simulink model "QCar2_Virtual_Car2"  (R2023a)
settings: Solver=ode1  StartTime=0.0  StopTime=inf  FixedStep=cameraStepSize/10  RelTol=1e-3  EnableMultiTasking=on
PreLoadFcn:
  | QCarSetup
values from neighbouring files (symbols this model uses):
  cameraStepSize = 3e-2    (= 0.03)    [QCarSetup.m]
  path_x = [0.826 0.836 0.846 0.856 0.866 0.876 0.886 0.896 0.906 0.916 0.926 0.936 ... (740 elements, 740x1)]    [SDTS_Paths_6_2023.mat]
  path_x2 = [-0.614 -0.604 -0.594 -0.584 -0.574 -0.564 -0.554 -0.544 -0.534 -0.524 -0.514 -0.504 ... (1090 elements, 1090x1)]    [SDTS_Paths_6_2023.mat]
  path_x3 = [-0.614 -0.603821428571 -0.593642857143 -0.583464285714 -0.573285714286 -0.563107142857 -0.552928571429 -0.54275 -0.532571428571 -0.522392857143 -0.512214285714 -0.502035714286 ... (714 elements, 714x1)]    [SDTS_Paths_6_2023.mat]
  path_x4 = [-0.614 -0.604 -0.594 -0.584 -0.574 -0.564 -0.554 -0.544 -0.534 -0.524 -0.514 -0.504 ... (1761 elements, 1761x1)]    [SDTS_Paths_6_2023.mat]
  path_x5 = [1.436 1.42588571429 1.41577142857 1.40565714286 1.39554285714 1.38542857143 1.37531428571 1.3652 1.35508571429 1.34497142857 1.33485714286 1.32474285714 ... (574 elements, 574x1)]    [SDTS_Paths_6_2023.mat]
  path_x6 = [1.436 1.42588571429 1.41577142857 1.40565714286 1.39554285714 1.38542857143 1.37531428571 1.3652 1.35508571429 1.34497142857 1.33485714286 1.32474285714 ... (1288 elements, 1288x1)]    [SDTS_Paths_6_2023.mat]
  path_y = [-1.0887 -1.0887 -1.0887 -1.0887 -1.0887 -1.0887 -1.0887 -1.0887 -1.0887 -1.0887 -1.0887 -1.0887 ... (740 elements, 740x1)]    [SDTS_Paths_6_2023.mat]
  path_y2 = [-1.0887 -1.0887 -1.0887 -1.0887 -1.0887 -1.0887 -1.0887 -1.0887 -1.0887 -1.0887 -1.0887 -1.0887 ... (1090 elements, 1090x1)]    [SDTS_Paths_6_2023.mat]
  path_y3 = [-1.0887 -1.0887 -1.0887 -1.0887 -1.0887 -1.0887 -1.0887 -1.0887 -1.0887 -1.0887 -1.0887 -1.0887 ... (714 elements, 714x1)]    [SDTS_Paths_6_2023.mat]
  path_y4 = [-1.0887 -1.0887 -1.0887 -1.0887 -1.0887 -1.0887 -1.0887 -1.0887 -1.0887 -1.0887 -1.0887 -1.0887 ... (1761 elements, 1761x1)]    [SDTS_Paths_6_2023.mat]
  path_y5 = [-0.8157 -0.8157 -0.8157 -0.8157 -0.8157 -0.8157 -0.8157 -0.8157 -0.8157 -0.8157 -0.8157 -0.8157 ... (574 elements, 574x1)]    [SDTS_Paths_6_2023.mat]
  path_y6 = [-0.8157 -0.8157 -0.8157 -0.8157 -0.8157 -0.8157 -0.8157 -0.8157 -0.8157 -0.8157 -0.8157 -0.8157 ... (1288 elements, 1288x1)]    [SDTS_Paths_6_2023.mat]
undefined symbols (not defined in the file or in its folder): DiscIntNeverNeededParam, gcbh, height, Host, JPEG, left, qc_get_step_size, top, video_display_show, width
libraries: quarc_library x71, simulink_extras x12, simulink x5
(part 1 of 5)
settings Model: SimulationMode=external  ExtModeTrigDuration=10000  Creator=user
settings SolverCC: AlgebraicLoopSolver=TrustRegion  PositivePriorityOrder=on
settings DataIOCC: ReturnWorkspaceOutputs=off
settings OptimizationCC: ReuseModelBlockBuffer=off
settings DebuggingCC: UnconnectedInputMsg=warning  UnconnectedOutputMsg=warning  UnconnectedLineMsg=warning  ArithmeticOperatorsInVariantConditions=warning
settings ModelReferenceCC: EnableRefExpFcnMdlSchedulingChecks=on
settings SFSimCC: SimUseLocalCustomCode=off  CustomCodeUndefinedFunction=UseInterfaceOnly
settings RTWCC: Description=QUARC Win64 Target Using Toolchain  SystemTargetFile=quarc_win64.tlc  TemplateMakefile=quarc_default_tmf  RTWUseLocalCustomCode=off  Toolchain=QUARC win64 | nmake (64-bit Windows)  BuildConfiguration=Faster Runs
settings CodeAppCC: StateflowObjectComments=on
settings STFCustomTargetCC: SystemTargetFile=quarc_win64.tlc
settings GRTTargetCC: ParMdlRefBuildCompliant=off  CompOptLevelCompliant=off  CombineOutputUpdateFcns=off  MatFileLogging=off  CPPClassGenCompliant=off  GRTInterface=on  ExtMode=on  ExtModeMexFile=quarc_comm
settings ConfigComp: CovMetricSettings=dswe

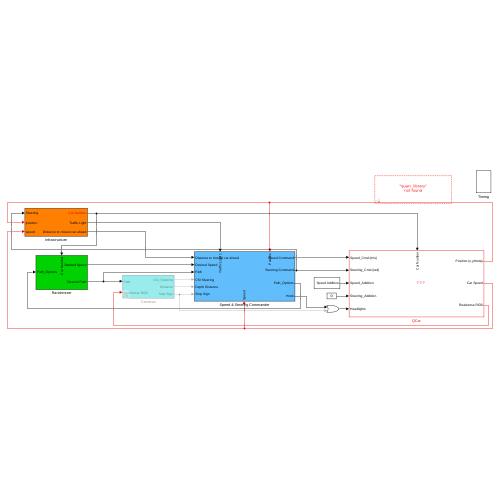
[thumbnail: Simulink's stored preview of the top-level diagram]
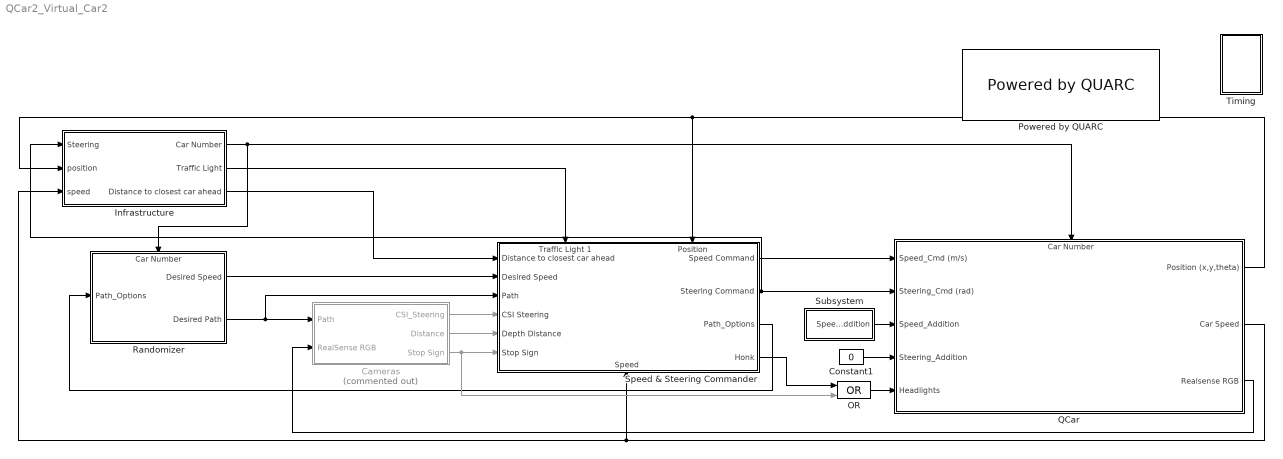
== system QCar2_Virtual_Car2 ==
  Cameras : Subsystem  Commented=on
  Constant1 : Constant  Value=0
  Infrastructure : Subsystem
  OR : Logic  Operator=OR  IconShape=distinctive  AllPortsSameDT=off  OutDataTypeStr=boolean
  Powered by QUARC : quarc_library/Logos/Powered by QUARC
  QCar : Subsystem
      settings: PortSchema="{\"entries\":[{\"content\":{\"sides\":[{\"content\":{\"connectorIds\":[\"In1\",\"In2\",\"In3\",\"In4\",\"In5\"]},\"type\":\"ConnectorPlacement.EquallySpacedRectSide\",\"uuid\":\"02a1560c-0405-4b97-a286-7d926425b90e\"},{\"content\":{\"connectorIds\":[\"Out1\",\"Out2\",\"Out3\"],\"side\":\"RIGHT\"},\"type\":\"ConnectorPlacement.EquallySpacedRectSide\",\"uuid\":\"39c5c8b2-4245-4ec7-b5b3-4c98e6a2673a\"},{\"content\":{\"connectorIds\":[\"In6\"],\"side\":\"TOP\"},\"type\":\"ConnectorPlacement.EquallySpacedRectSide\",\"uuid\":\"1752f2f8-f0ed-4d28-b225-c74112047425\"}]},\"type\":\"ConnectorPlacement.EquallySpacedConnector\",\"uuid\":\"d58cf7e2-2005-4c93-8747-d53ee0601380\"}],\"packageUris\":[\"http://schema.mathworks.com/mf0/Connector/R2020b\"],\"version\":\"1.0\"}"
      mask Display: image('QCar.png'); % Use "Edit Image" on toolstrip to change.
  Randomizer : Subsystem
      settings: PortSchema="{\"entries\":[{\"content\":{\"sides\":[{\"content\":{\"connectorIds\":[\"In1\"]},\"type\":\"ConnectorPlacement.EquallySpacedRectSide\",\"uuid\":\"79c25646-074c-450f-bb45-0d8852c7e7f6\"},{\"content\":{\"connectorIds\":[\"Out1\",\"Out2\"],\"side\":\"RIGHT\"},\"type\":\"ConnectorPlacement.EquallySpacedRectSide\",\"uuid\":\"212c2e10-164c-43b0-8e79-58f131c612df\"},{\"content\":{\"connectorIds\":[\"In2\"],\"side\":\"TOP\"},\"type\":\"ConnectorPlacement.EquallySpacedRectSide\",\"uuid\":\"61fd9557-f0fe-45db-bcdc-894cad4630c6\"}]},\"type\":\"ConnectorPlacement.EquallySpacedConnector\",\"uuid\":\"547c8944-af2b-4298-88bf-ccf6c0f693d3\"}],\"packageUris\":[\"http://schema.mathworks.com/mf0/Connector/R2020b\"],\"version\":\"1.0\"}"
  Speed & Steering Commander : Subsystem
      settings: PortSchema="{\"entries\":[{\"content\":{\"sides\":[{\"content\":{\"connectorIds\":[\"In1\",\"In2\",\"In3\",\"In4\",\"In5\",\"In6\"]},\"type\":\"ConnectorPlacement.EquallySpacedRectSide\",\"uuid\":\"9b63f585-0ce9-4b0b-9aa1-11e6ffafcd91\"},{\"content\":{\"connectorIds\":[\"Out1\",\"Out2\",\"Out3\",\"Out4\"],\"side\":\"RIGHT\"},\"type\":\"ConnectorPlacement.EquallySpacedRectSide\",\"uuid\":\"3f0be152-fc9f-4953-a169-b2152976c976\"},{\"content\":{\"connectorIds\":[\"In7\",\"In8\"],\"side\":\"TOP\"},\"type\":\"ConnectorPlacement.EquallySpacedRectSide\",\"uuid\":\"393ea782-c0f7-40ad-a810-9b99db6be290\"},{\"content\":{\"connectorIds\":[\"In9\"],\"side\":\"BOTTOM\"},\"type\":\"ConnectorPlacement.EquallySpacedRectSide\",\"uuid\":\"5db59a4e-a267-4a7e-baba-ee9e0de1ecf8\"}]},\"type\":\"ConnectorPlacement.EquallySpacedConnector\",\"uuid\":\"cc2e920a-311c-4c49-a19e-cf12c76a97eb\"}],\"packageUris\":[\"http://schema.mathworks.com/mf0/Connector/R2020b\"],\"version\":\"1.0\"}"
  Subsystem : Subsystem
  Timing : Subsystem
  wires:
  Infrastructure/2(Traffic Light) -> Speed & Steering Commander/7(Traffic Light 1)
  Speed & Steering Commander/4(Honk) -> OR/1
  OR/1 -> QCar/5(Headlights)
  QCar/3(Realsense RGB) -> Cameras/2(RealSense RGB)
  QCar/2(Car Speed) -> Infrastructure/3("speed "), Speed & Steering Commander/9(Speed)
  Speed & Steering Commander/3(Path_Options) -> Randomizer/1(Path_Options)
  Cameras/3(Stop Sign) -> OR/2, Speed & Steering Commander/6(Stop Sign)
  Randomizer/2(Desired Path) -> Speed & Steering Commander/3(Path), Cameras/1(Path)
  Infrastructure/1(Car Number) -> QCar/6(Car Number), Randomizer/2(Car Number)
  Cameras/2(Distance) -> Speed & Steering Commander/5(Depth Distance)
  Speed & Steering Commander/1(Speed Command) -> QCar/1(Speed_Cmd (m/s))
  QCar/1(Position (x,y,theta)) -> Speed & Steering Commander/8(Position), Infrastructure/2(position)
  Infrastructure/3(Distance to closest car ahead) -> Speed & Steering Commander/1(Distance to closest car ahead)
  Cameras/1(CSI_Steering) -> Speed & Steering Commander/4(CSI Steering)
  Speed & Steering Commander/2(Steering Command) -> Infrastructure/1(Steering), QCar/2(Steering_Cmd (rad))
  Constant1/1 -> QCar/4(Steering_Addition)
  Randomizer/1(Desired Speed) -> Speed & Steering Commander/2(Desired Speed)
  Subsystem/1(Speed Addition) -> QCar/3(Speed_Addition)

== system QCar2_Virtual_Car2/Cameras ==
  Path : Inport
  RealSense RGB : Inport  Port=2
  CSI Camera : Subsystem  Commented=on
  Classifier : Scope
  Demux : Demux  Outputs=5
  Goto : Goto  Commented=on  GotoTag=CSI_Steering
  Goto1 : Goto  Commented=on  GotoTag=CSI_Score
  Goto23 : Goto  Commented=on  GotoTag=Found_Lane
  Goto24 : Goto  Commented=on  GotoTag=Lost_Lane
  Image Transform : quarc_library/Image Processing/Generic/Image Transform  algorithm=Resize  color_theme=KRYGCBMW  min_pixel=0  max_pixel=4000  contour_depth=1  focal_length=308  principal_point=[262 334]  radial_coeffs=[-0.3129 0.0907]  tangential_coeffs=[]  extrapolated_pixel=0  interpolation=nearest  row_coords=0  column_coords=0  output_height=224  output_width=224  angle=0  origin=[240 320]  output_origin=[240 320]  output_data_type=uint8
      settings: AttributesFormatString=(%<algorithm>)  SourceProductName=QUARC Targets
  Rate Transition : RateTransition
  Real Sense : Subsystem  LoadFcn=set_param(gcbh, 'UserData', gcb);  StartFcn=video_display_show([gcb, '/Video Display'], 'add', gcb);  mask(Video Compressed Display){algorithm=JPEG, quality=50, sample_time=-1, use_hardware=on}
      mask prompts: algorithm "Compression algorithm:"; quality "Compression quality (0-100):"; sample_time "Sample time (seconds):"; use_hardware "Use hardware acceleration for video display"
      mask help: Displays a video stream on the host, using compression to minimize bandwidth.
      mask init:
      | qc_set_display('Video\nCompressed\nDisplay');
      settings: UndoDeleteFcn=set_param(gcbh, 'UserData', gcb);  OpenFcn=video_display_show([gcb, '/Video Display'], 'show', gcb);  PreDeleteFcn=video_display_show([gcb, '/Video Display'], 'delete');
      settings: CopyFcn=|
      | set_param(gcbh, 'UserData', gcb);
      | set_param(gcbh, 'LinkStatus', 'none');
      settings: NameChangeFcn=|
      | video_display_show([get_param(gcbh, 'UserData'), '/Video Display'], 'rename', [gcb, '/Video Display']);
      | video_display_show([gcb, '/Video Display'], 'add', gcb);
      | set_param(gcbh, 'UserData', gcb);
      mask Help: web(qc_get_block_help_path(gcb));
      mask TypeOptions algorithm: Image Compress/algorithm
      mask TypeOptions quality: Image Compress/quality
      mask TypeOptions sample_time: Video Display/sample_time
      mask TypeOptions use_hardware: Video Display/use_hardware
      mask Display:
      | patch([0.98591 0.98591 0.62618 0.59072 0.56147   0.536   0.536  0.5441 0.56912 0.59207 0.60881 0.62276 0.63527 0.64364  0.6485  0.6485 0.64706 0.64499 0.63662 0.62411 0.61232 0.59837 0.58307 0.56147   0.536   0.536  0.5441  0.5747 0.60953 0.63662 0.67001  0.7034 0.72851 0.75425 0.77927 0.80294 0.82454 0.84119 0.85865 0.87395 0.88574 0.89339  0.8969 0.89969 0.89969 0.89267  0.8816 0.87044 0.85649  0.8384 0.81824 0.80294 0.78764 0.77513 0.76676 0.75776 0.76397 0.77513 0.79178 0.80987 0.82796 0.84326 0.86207 0.98528],[0.18689 0.05522 0.05522 0.05171 0.05171    0.05 0.18338 0.18338 0.19148 0.20435 0.22298 0.24863 0.28589 0.33125 0.38138 0.55139 0.59801 0.63761 0.68189 0.72149 0.74939 0.76694 0.77855 0.79367 0.79952 0.92768 0.92768 0.92768 0.92417 0.92066 0.91364  0.9032 0.89384 0.88106 0.86594 0.85073 0.82634 0.80537 0.77855 0.74363 0.70403 0.65858 0.61079 0.59099 0.41513 0.37202 0.31847 0.29048 0.25556 0.23342  0.2102 0.19382 0.18221 0.17285 0.16943 0.16124  0.1589 0.16241 0.16709 0.17168  0.1787 0.18221 0.18689 0.18689],[0.9,0.90,0.91])
      | patch([0.536 0.52601 0.46823 0.44528 0.41603 0.39101 0.35555 0.33116 0.31451 0.29291  0.2804 0.26717 0.25322 0.23999 0.22406 0.20732 0.19337 0.17528 0.15935 0.14396 0.13217 0.11759 0.10922 0.10085 0.09671 0.09392 0.09041 0.08906 0.08906 0.09464  0.0995 0.10778 0.11894 0.13145 0.14675 0.16349 0.17672 0.19409 0.20732 0.22406 0.23999 0.26159 0.27833 0.29849 0.31793 0.33602 0.35411 0.37085 0.39245 0.41603   0.536   0.536 0.53159 0.46409   0.446 0.42026 0.39587 0.37571 0.36113 0.34925 0.34088 0.33809 0.33809 0.34088 0.34583 0.35627 0.36392 0.38129 0.39587 0.41117 0.42719 0.44672  0.4676 0.48353 0.48353 0.52394   0.536],[0.05 0.04829 0.04712 0.04712 0.04829 0.05063 0.05405 0.05873 0.06107 0.06692 0.07043 0.07619 0.08087 0.08672 0.09482 0.10652 0.11696 0.13325  0.1508 0.17168 0.19499 0.22415 0.25439 0.28472 0.31379 0.35456 0.38489 0.41513 0.58055 0.63878 0.68774 0.72149 0.75641 0.78089 0.80537 0.82859 0.84029 0.85658 0.86594 0.87404  0.8834 0.89267 0.90086 0.90788 0.91247 0.91832 0.92066   0.923 0.92651 0.92768 0.92768 0.79952 0.79952 0.79952 0.79718 0.78899 0.77153 0.75056 0.72149 0.68072 0.62249  0.5549 0.41396 0.37085 0.33242 0.28121 0.25205 0.22181 0.20552 0.19499 0.18572 0.18221 0.17753 0.17636 0.17753  0.1787  0.1787],[0.9,0.90,0.91])
      | disp('Video\nCompressed\nDisplay');
  S-Function : S-Function  Commented=on  FunctionName=classify_image_caller  SFunctionDeploymentMode=off  EnableBusSupport=off
  Selector : Selector  NumberOfDimensions=3  InputPortWidth=3  IndexOptions=Select all,Index vector (dialog),Select all  Indices=[1 3],140:499,1  OutputSizes=1,1,1
  Sign Finder : Subsystem
  Sign ROI : Subsystem  LoadFcn=set_param(gcbh, 'UserData', gcb);  StartFcn=video_display_show([gcb, '/Video Display'], 'add', gcb);  mask(Video Compressed Display){algorithm=JPEG, quality=50, sample_time=-1, use_hardware=on}
      mask prompts: algorithm "Compression algorithm:"; quality "Compression quality (0-100):"; sample_time "Sample time (seconds):"; use_hardware "Use hardware acceleration for video display"
      mask help: Displays a video stream on the host, using compression to minimize bandwidth.
      mask init:
      | qc_set_display('Video\nCompressed\nDisplay');
      settings: UndoDeleteFcn=set_param(gcbh, 'UserData', gcb);  OpenFcn=video_display_show([gcb, '/Video Display'], 'show', gcb);  PreDeleteFcn=video_display_show([gcb, '/Video Display'], 'delete');
      settings: CopyFcn=|
      | set_param(gcbh, 'UserData', gcb);
      | set_param(gcbh, 'LinkStatus', 'none');
      settings: NameChangeFcn=|
      | video_display_show([get_param(gcbh, 'UserData'), '/Video Display'], 'rename', [gcb, '/Video Display']);
      | video_display_show([gcb, '/Video Display'], 'add', gcb);
      | set_param(gcbh, 'UserData', gcb);
      mask Help: web(qc_get_block_help_path(gcb));
      mask TypeOptions algorithm: Image Compress/algorithm
      mask TypeOptions quality: Image Compress/quality
      mask TypeOptions sample_time: Video Display/sample_time
      mask TypeOptions use_hardware: Video Display/use_hardware
      mask Display:
      | patch([0.98591 0.98591 0.62618 0.59072 0.56147   0.536   0.536  0.5441 0.56912 0.59207 0.60881 0.62276 0.63527 0.64364  0.6485  0.6485 0.64706 0.64499 0.63662 0.62411 0.61232 0.59837 0.58307 0.56147   0.536   0.536  0.5441  0.5747 0.60953 0.63662 0.67001  0.7034 0.72851 0.75425 0.77927 0.80294 0.82454 0.84119 0.85865 0.87395 0.88574 0.89339  0.8969 0.89969 0.89969 0.89267  0.8816 0.87044 0.85649  0.8384 0.81824 0.80294 0.78764 0.77513 0.76676 0.75776 0.76397 0.77513 0.79178 0.80987 0.82796 0.84326 0.86207 0.98528],[0.18689 0.05522 0.05522 0.05171 0.05171    0.05 0.18338 0.18338 0.19148 0.20435 0.22298 0.24863 0.28589 0.33125 0.38138 0.55139 0.59801 0.63761 0.68189 0.72149 0.74939 0.76694 0.77855 0.79367 0.79952 0.92768 0.92768 0.92768 0.92417 0.92066 0.91364  0.9032 0.89384 0.88106 0.86594 0.85073 0.82634 0.80537 0.77855 0.74363 0.70403 0.65858 0.61079 0.59099 0.41513 0.37202 0.31847 0.29048 0.25556 0.23342  0.2102 0.19382 0.18221 0.17285 0.16943 0.16124  0.1589 0.16241 0.16709 0.17168  0.1787 0.18221 0.18689 0.18689],[0.9,0.90,0.91])
      | patch([0.536 0.52601 0.46823 0.44528 0.41603 0.39101 0.35555 0.33116 0.31451 0.29291  0.2804 0.26717 0.25322 0.23999 0.22406 0.20732 0.19337 0.17528 0.15935 0.14396 0.13217 0.11759 0.10922 0.10085 0.09671 0.09392 0.09041 0.08906 0.08906 0.09464  0.0995 0.10778 0.11894 0.13145 0.14675 0.16349 0.17672 0.19409 0.20732 0.22406 0.23999 0.26159 0.27833 0.29849 0.31793 0.33602 0.35411 0.37085 0.39245 0.41603   0.536   0.536 0.53159 0.46409   0.446 0.42026 0.39587 0.37571 0.36113 0.34925 0.34088 0.33809 0.33809 0.34088 0.34583 0.35627 0.36392 0.38129 0.39587 0.41117 0.42719 0.44672  0.4676 0.48353 0.48353 0.52394   0.536],[0.05 0.04829 0.04712 0.04712 0.04829 0.05063 0.05405 0.05873 0.06107 0.06692 0.07043 0.07619 0.08087 0.08672 0.09482 0.10652 0.11696 0.13325  0.1508 0.17168 0.19499 0.22415 0.25439 0.28472 0.31379 0.35456 0.38489 0.41513 0.58055 0.63878 0.68774 0.72149 0.75641 0.78089 0.80537 0.82859 0.84029 0.85658 0.86594 0.87404  0.8834 0.89267 0.90086 0.90788 0.91247 0.91832 0.92066   0.923 0.92651 0.92768 0.92768 0.79952 0.79952 0.79952 0.79718 0.78899 0.77153 0.75056 0.72149 0.68072 0.62249  0.5549 0.41396 0.37085 0.33242 0.28121 0.25205 0.22181 0.20552 0.19499 0.18572 0.18221 0.17753 0.17636 0.17753  0.1787  0.1787],[0.9,0.90,0.91])
      | disp('Video\nCompressed\nDisplay');
  Stop : Scope
  Stop1 : Scope
  CSI_Steering : Outport
  Distance : Outport  Port=2
  Stop Sign : Outport  Port=3
  wires:
  Selector/1 -> Image Transform/1
  Sign Finder/1(Stop Sign) -> Stop/1, Stop Sign/1
  Demux/4 -> Stop1/1
  RealSense RGB/1 -> Selector/1, Real Sense/1(In1)
  S-Function/1 -> Rate Transition/1, Classifier/1, Demux/1
  Image Transform/1 -> S-Function/1, Sign ROI/1(In1)
  Rate Transition/1 -> Sign Finder/1(Signs)
  CSI Camera/3(Found Lane) -> Goto23/1
  CSI Camera/1(Steering) -> Goto/1, CSI_Steering/1
  CSI Camera/2(Score) -> Goto1/1
  CSI Camera/4(Lost Lane) -> Goto24/1

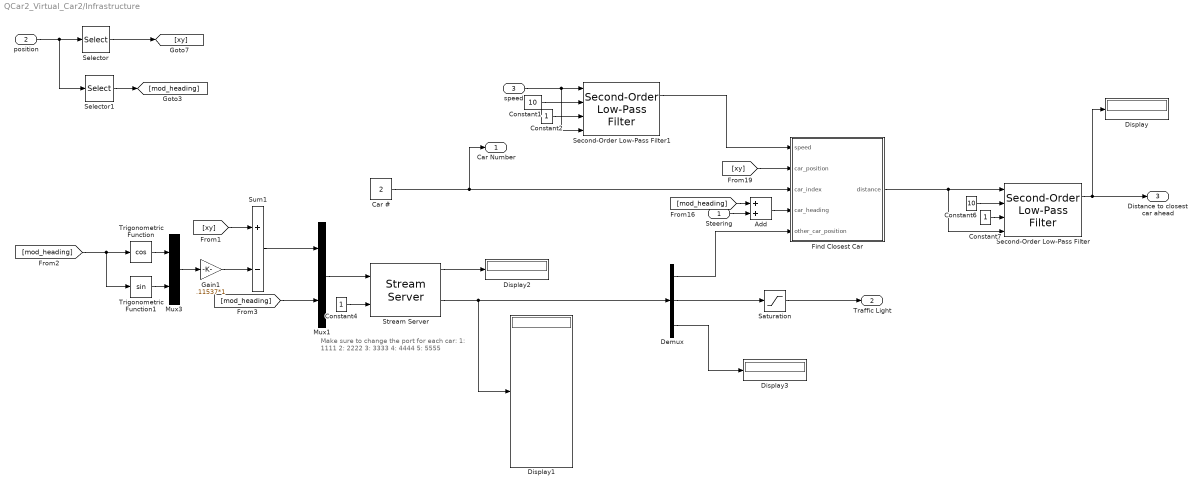
== system QCar2_Virtual_Car2/Infrastructure ==
  note: Make sure to change the port for each car:
      | 1: 1111
      | 2: 2222
      | 3: 3333
      | 4: 4444
      | 5: 5555
  Steering : Inport
  position : Inport  Port=2
  "speed " : Inport  Port=3
  Add : Sum
  Car # : Constant  Value=2
  Constant1 : Constant  Value=10
  Constant2 : Constant
  Constant4 : Constant
  Constant6 : Constant  Value=10
  Constant7 : Constant
  Demux : Demux  Outputs=[10 1 1]
  Display{,1..3} (4 alike) : Display
      Display2 settings: Decimation=100
      Display3 settings: Decimation=100
  Find Closest Car : Subsystem
  Gain1 : Gain  Gain=.11537*1
  Mux1 : Mux  Inputs=2
  Mux3 : Mux  Inputs=2
  Saturation : Saturate  UpperLimit=1  LowerLimit=0
  Second-Order Low-Pass Filter : quarc_library/Continuous/Second-Order Low-Pass Filter  params_source=External (input ports)  input_width=1  input_zeta=1  input_init=0
  Second-Order Low-Pass Filter1 : quarc_library/Continuous/Second-Order Low-Pass Filter  params_source=External (input ports)  input_width=1  input_zeta=1  input_init=0
  Selector : Selector  InputPortWidth=3  IndexOptions=Index vector (dialog)  Indices=1:2  OutputSizes=1
  Selector1 : Selector  InputPortWidth=3  IndexOptions=Index vector (dialog)  Indices=3  OutputSizes=1
  Stream Server : quarc_library/Communications/Basic/Stream Server  uri_source=Specify via dialog (do not evaluate)  uri=tcpip://localhost:2222  send_buffer_size=1460  receive_buffer_size=1460  byte_order=little endian (Intel - LSB first)  optimization=Minimum latency  send_options=Send most recent data  receive_options=Receive most recent data  default_value=10* ones (1,12)  sample_time=qc_get_step_size  active=off  implementation=Use blocking I/O in a separate thread  send_fifo_size=1000  receive_fifo_size=1000  send_priority=0  receive_priority=0  send_dimensions=off  receive_dimensions=off  max_dimensions=-1  data_type=Inherited via back propagation  type_expr=BusObject
      settings: AttributesFormatString="\"tcpip://localhost:2222\""
  Sum1 : Sum  Inputs=+-
  Trigonometric Function : Trigonometry  Operator=cos
  Trigonometric Function1 : Trigonometry
  Car Number : Outport
  Traffic Light : Outport  Port=2
  Distance to closest car ahead : Outport  Port=3
  wires:
  Mux1/1 -> Stream Server/1
  [xy] -> Sum1/1
  Mux3/1 -> Gain1/1
  Trigonometric Function1/1 -> Mux3/2
  Trigonometric Function/1 -> Mux3/1
  Gain1/1 -> Sum1/2
  Saturation/1 -> Traffic Light/1
  Demux/2 -> Saturation/1
  Demux/1 -> Find Closest Car/5(other_car_position)
  Steering/1 -> Add/2
  [mod_heading] -> Add/1
  Add/1 -> Find Closest Car/4(car_heading)
  Find Closest Car/1(distance) -> Second-Order Low-Pass Filter/1, Second-Order Low-Pass Filter/4
  Second-Order Low-Pass Filter1/1 -> Find Closest Car/1("speed ")
  Constant2/1 -> Second-Order Low-Pass Filter1/3
  [xy] -> Find Closest Car/2(car_position)
  "speed "/1 -> Second-Order Low-Pass Filter1/1, Second-Order Low-Pass Filter1/4
  Car #/1 -> Car Number/1, Find Closest Car/3(car_index)
  Constant1/1 -> Second-Order Low-Pass Filter1/2
  Second-Order Low-Pass Filter/1 -> Distance to closest car ahead/1, Display/1
  Selector1/1 -> [mod_heading]
  Selector/1 -> [xy]
  position/1 -> Selector/1, Selector1/1
  Constant6/1 -> Second-Order Low-Pass Filter/2
  Constant4/1 -> Stream Server/2
  Constant7/1 -> Second-Order Low-Pass Filter/3
  Stream Server/1 -> Display2/1
  Stream Server/4 -> Display1/1, Demux/1
  Sum1/1 -> Mux1/1
  [mod_heading] -> Mux1/2
  [mod_heading] -> Trigonometric Function1/1, Trigonometric Function/1
  Demux/3 -> Display3/1

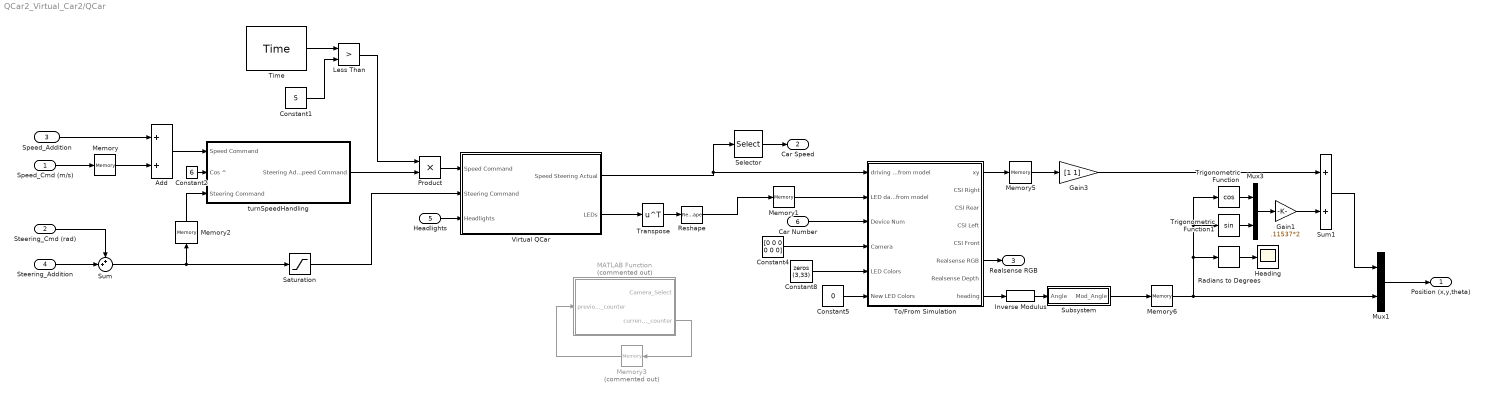
== system QCar2_Virtual_Car2/QCar ==
  Speed_Cmd (m/s) : Inport
  Steering_Cmd (rad) : Inport  Port=2
  Speed_Addition : Inport  Port=3
  Steering_Addition : Inport  Port=4
  Headlights : Inport  Port=5
  Car Number : Inport  Port=6
  Add : Sum
  Constant1 : Constant  Value=5
  Constant2 : Constant  Value=6
  Constant4 : Constant  Value=[0 0 0 0 0 0]
  Constant5 : Constant  Value=0
  Constant8 : Constant  Value=zeros (3,33)
  Gain1 : Gain  Gain=.11537*2
  Gain3 : Gain  Gain=[1 1]
  Heading : Scope
  Inverse Modulus : quarc_library/Discontinuities/Inverse Modulus  modulus=2*pi  output_derivative=off  output_revolutions=off  max_x=Inf  min_x=-Inf
  Less Than : RelationalOperator  Operator=>  OutDataTypeStr=boolean  RndMeth=Simplest  InputSameDT=off
  MATLAB Function : MATLAB Function  Commented=on  TreatAsAtomicUnit=on
  Memory : Memory  InheritSampleTime=on  LinearizeMemory=on  LinearizeAsDelay=on
  Memory1 : Memory  InitialCondition=zeros (1,16)  InheritSampleTime=on  LinearizeMemory=on  LinearizeAsDelay=on
  Memory2 : Memory  InheritSampleTime=on  LinearizeMemory=on  LinearizeAsDelay=on
  Memory3 : Memory  Commented=on  InheritSampleTime=on  LinearizeMemory=on  LinearizeAsDelay=on
  Memory5 : Memory  InitialCondition=[0 0]  InheritSampleTime=on  LinearizeMemory=on  LinearizeAsDelay=on
  Memory6 : Memory  InheritSampleTime=on  LinearizeMemory=on  LinearizeAsDelay=on
  Mux1 : Mux  Inputs=2
  Mux3 : Mux  Inputs=2
  Product : Product
  Radians to Degrees : simulink_extras/Transformations/Radians to Degrees
  Reshape : Reshape
  Saturation : Saturate  UpperLimit=0.6  LowerLimit=-0.6
  Selector : Selector  InputPortWidth=2  IndexOptions=Index vector (dialog)  Indices=[1]  OutputSizes=1
  Subsystem : Subsystem
  Sum : Sum  Inputs=++|
  Sum1 : Sum
  Time : quarc_library/Sources/Time/Time  time_source=Wall clock  sample_time=qc_get_step_size
  To/From Simulation : Subsystem
  Transpose : Math  Operator=transpose
  Trigonometric Function : Trigonometry  Operator=cos
  Trigonometric Function1 : Trigonometry
  Virtual QCar : Subsystem
  turnSpeedHandling : Subsystem
  Position (x,y,theta) : Outport
  Car Speed : Outport  Port=2
  Realsense RGB : Outport  Port=3
  wires:
  Saturation/1 -> Virtual QCar/2(Steering Command)
  Memory6/1 -> Mux1/2, Trigonometric Function/1, Trigonometric Function1/1, Radians to Degrees/1
  Subsystem/1(Mod_Angle) -> Memory6/1
  Memory5/1 -> Gain3/1
  Headlights/1 -> Virtual QCar/3(Headlights)
  Memory3/1 -> MATLAB Function/1(previous_counter)
  MATLAB Function/2(current_counter) -> Memory3/1
  Mux1/1 -> Position (x,y,theta)/1
  Sum1/1 -> Mux1/1
  Memory2/1 -> turnSpeedHandling/3(Steering Command)
  Add/1 -> turnSpeedHandling/1(Speed Command)
  Constant2/1 -> turnSpeedHandling/2(Cos ^)
  Car Number/1 -> To/From Simulation/3(Device Num)
  Gain3/1 -> Sum1/1
  Gain1/1 -> Sum1/2
  Mux3/1 -> Gain1/1
  Trigonometric Function1/1 -> Mux3/2
  Trigonometric Function/1 -> Mux3/1
  Sum/1 -> Saturation/1, Memory2/1
  Steering_Addition/1 -> Sum/2
  Radians to Degrees/1 -> Heading/1
  Memory/1 -> Add/2
  Steering_Cmd (rad)/1 -> Sum/1
  Speed_Cmd (m/s)/1 -> Memory/1
  Speed_Addition/1 -> Add/1
  Inverse Modulus/1 -> Subsystem/1(Angle)
  Virtual QCar/1(Speed Steering Actual) -> Selector/1, To/From Simulation/1(driving data from model)
  Selector/1 -> Car Speed/1
  Constant4/1 -> To/From Simulation/4(Camera)
  Constant8/1 -> To/From Simulation/5(LED Colors)
  Constant5/1 -> To/From Simulation/6(New LED Colors)
  To/From Simulation/8(heading) -> Inverse Modulus/1
  To/From Simulation/1(xy) -> Memory5/1
  To/From Simulation/6(Realsense RGB) -> Realsense RGB/1
  Memory1/1 -> To/From Simulation/2(LED data from model)
  Virtual QCar/2(LEDs) -> Transpose/1
  Transpose/1 -> Reshape/1
  Reshape/1 -> Memory1/1
  Time/1 -> Less Than/1
  Constant1/1 -> Less Than/2
  Less Than/1 -> Product/1
  Product/1 -> Virtual QCar/1(Speed Command)
  turnSpeedHandling/1(Steering Adjusted Speed Command) -> Product/2

== system QCar2_Virtual_Car2/Randomizer ==
  Path_Options : Inport
  Car Number : Inport  Port=2
  Constant1 : Constant  Value=.75
  Constant2 : Constant
  Constant3 : Constant  Value=2
  Constant4 : Constant  Value=2
  Constant5 : Constant  Value=0.7
  Constant6 : Constant  Value=0.4
  Constant7 : Constant  Value=0
  Display : Display
  Display1 : Display
  Display2 : Display
  MATLAB Function : MATLAB Function  TreatAsAtomicUnit=on
  Manual Switch : ManualSwitch
  Manual Switch1 : ManualSwitch
  Manual Switch2 : ManualSwitch
  Memory1 : Memory  InitialCondition=2  InheritSampleTime=on  LinearizeMemory=on  LinearizeAsDelay=on
  Memory2 : Memory  InitialCondition=1  InheritSampleTime=on  LinearizeMemory=on  LinearizeAsDelay=on
  Multiport Switch : MultiPortSwitch  SaturateOnIntegerOverflow=off  InputSameDT=off
  Subsystem1 : Subsystem
  Desired Speed : Outport
  Desired Path : Outport  Port=2
  wires:
  Path_Options/1 -> MATLAB Function/3(Path_Options), Display2/1
  Manual Switch2/1 -> Desired Path/1
  Constant4/1 -> Manual Switch2/2
  Manual Switch/1 -> MATLAB Function/4(Speed_Cmd_Base)
  Constant1/1 -> Manual Switch/1
  Subsystem1/1(RisingEdgeTrigger) -> MATLAB Function/5(randomize)
  Constant3/1 -> Subsystem1/1(Random Period)
  MATLAB Function/2(Desired_Speed) -> Display1/1, Memory2/1
  MATLAB Function/1(Desired_Path) -> Display/1, Manual Switch2/1, Memory1/1
  Memory2/1 -> MATLAB Function/2(Previous_Speed)
  Memory1/1 -> MATLAB Function/1(Previous_Path)
  Car Number/1 -> Multiport Switch/1
  Constant2/1 -> Multiport Switch/2
  Constant5/1 -> Multiport Switch/3
  Constant6/1 -> Multiport Switch/4
  Multiport Switch/1 -> Manual Switch1/1
  Manual Switch1/1 -> Desired Speed/1
  Constant7/1 -> Manual Switch1/2

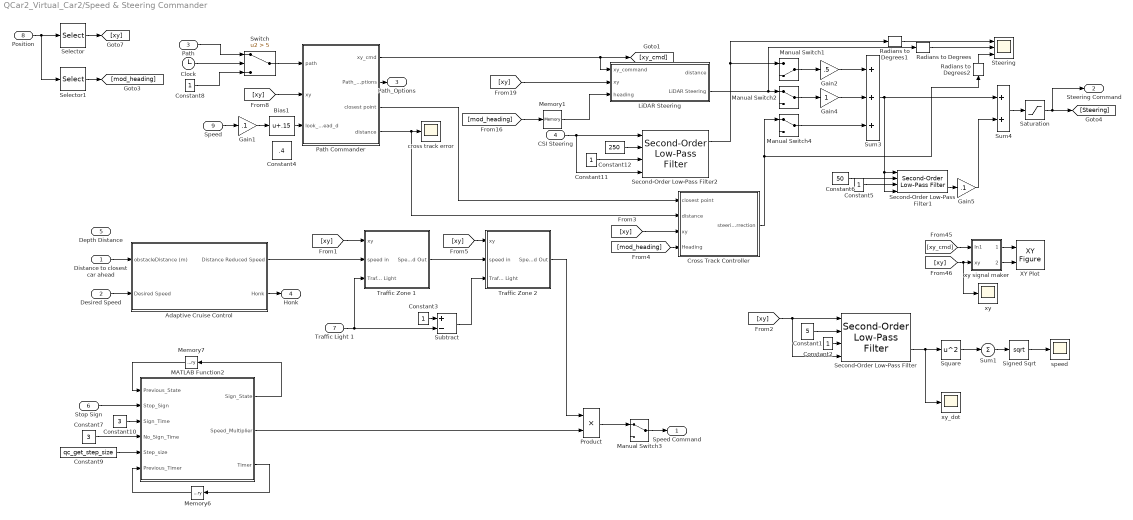
== system QCar2_Virtual_Car2/Speed & Steering Commander ==
  Distance to closest car ahead : Inport
  Desired Speed : Inport  Port=2
  Path : Inport  Port=3
  CSI Steering : Inport  Port=4
  Depth Distance : Inport  Port=5
  Stop Sign : Inport  Port=6
  Traffic Light 1 : Inport  Port=7
  Position : Inport  Port=8
  Speed : Inport  Port=9
  Adaptive Cruise Control : Subsystem
  Bias1 : Bias  Bias=.15  SaturateOnIntegerOverflow=off
  Clock : Clock
  Constant1 : Constant  Value=5
  Constant10 : Constant  Value=3
  Constant{2..3,5,8,11} (5 alike) : Constant
  Constant12 : Constant  Value=250
  Constant4 : Constant  Value=.4
  Constant6 : Constant  Value=50
  Constant7 : Constant  Value=3
  Constant9 : Constant  Value=qc_get_step_size
  Cross Track Controller : Subsystem
  Gain1 : Gain  Gain=.1
  Gain2 : Gain  Gain=.5
  Gain4 : Gain
  Gain5 : Gain  Gain=.1
  LiDAR Steering : Subsystem
  MATLAB Function2 : MATLAB Function  TreatAsAtomicUnit=on
  Manual Switch1 : ManualSwitch  CurrentSetting=0
  Manual Switch2 : ManualSwitch
  Manual Switch3 : ManualSwitch
  Manual Switch4 : ManualSwitch
  Memory1 : Memory
  Memory6 : Memory  InheritSampleTime=on  LinearizeMemory=on  LinearizeAsDelay=on
  Memory7 : Memory  InitialCondition=1  InheritSampleTime=on  LinearizeMemory=on  LinearizeAsDelay=on
  Path Commander : Subsystem
  Product : Product
  Radians to Degrees : simulink_extras/Transformations/Radians to Degrees
  Radians to Degrees1 : simulink_extras/Transformations/Radians to Degrees
  Radians to Degrees2 : simulink_extras/Transformations/Radians to Degrees
  Saturation : Saturate  UpperLimit=.6  LowerLimit=-0.6
  Second-Order Low-Pass Filter : quarc_library/Continuous/Second-Order Low-Pass Filter  params_source=External (input ports)  input_width=1  input_zeta=1  input_init=0
  Second-Order Low-Pass Filter1 : quarc_library/Continuous/Second-Order Low-Pass Filter  params_source=External (input ports)  input_width=1  input_zeta=1  input_init=0
  Second-Order Low-Pass Filter2 : quarc_library/Continuous/Second-Order Low-Pass Filter  params_source=External (input ports)  input_width=1  input_zeta=1  input_init=0
  Selector : Selector  InputPortWidth=3  IndexOptions=Index vector (dialog)  Indices=1:2  OutputSizes=1
  Selector1 : Selector  InputPortWidth=3  IndexOptions=Index vector (dialog)  Indices=3  OutputSizes=1
  Signed Sqrt : Sqrt
  Square : Math  Operator=square
  Steering : Scope  NumInputPorts=3
  Subtract : Sum  Inputs=+-
  Sum1 : Sum  Inputs=+
  Sum3 : Sum  Inputs=+++
  Sum4 : Sum
  Switch : Switch  Criteria=u2 > Threshold  Threshold=5  SaturateOnIntegerOverflow=off  InputSameDT=off
  Traffic Zone 1 : Subsystem
  Traffic Zone 2 : Subsystem
  XY Plot : quarc_library/Sinks/Figures/XY Figure  figure_mode=Use figure window  figure_tag=figure1  axes_tag=axes1  plot_mode=Time-based  minimum_x=-5  maximum_x=5  minimum_y=-2  maximum_y=5  buffer_size=1e3  update_rate=20  initial_position="1922     2   958  1021"  initial_visibility=on  sample_time=-1
      settings: SourceProductName=QUARC Targets
  cross track error : Scope
  speed : Scope
  xy : Scope
  xy signal maker : Subsystem
  xy_dot : Scope
  Speed Command : Outport
  Steering Command : Outport  Port=2
  Path_Options : Outport  Port=3
  Honk : Outport  Port=4
  wires:
  Memory1/1 -> LiDAR Steering/3(heading)
  [xy] -> LiDAR Steering/2(xy)
  Adaptive Cruise Control/2(Honk) -> Honk/1
  Constant3/1 -> Subtract/1
  Traffic Zone 2/1(Speed Out) -> Product/1
  Traffic Zone 1/1(Speed Out) -> Traffic Zone 2/2(speed in)
  [xy] -> Traffic Zone 2/1(xy)
  Adaptive Cruise Control/1(Distance Reduced Speed) -> Traffic Zone 1/2(speed in)
  Path Commander/4(distance) -> Cross Track Controller/2(distance), cross track error/1
  Cross Track Controller/1(steering correction) -> Manual Switch4/1, Radians to Degrees2/1
  Manual Switch4/1 -> Sum3/3
  [mod_heading] -> Cross Track Controller/4(Heading)
  [xy] -> Cross Track Controller/3(xy)
  Path Commander/3(closest point) -> Cross Track Controller/1(closest point)
  Manual Switch3/1 -> Speed Command/1
  Product/1 -> Manual Switch3/1
  [xy] -> Traffic Zone 1/1(xy)
  Constant12/1 -> Second-Order Low-Pass Filter2/2
  Constant11/1 -> Second-Order Low-Pass Filter2/3
  Second-Order Low-Pass Filter2/1 -> Manual Switch1/1, Radians to Degrees1/1
  CSI Steering/1 -> Second-Order Low-Pass Filter2/4, Second-Order Low-Pass Filter2/1
  Radians to Degrees2/1 -> Steering/3
  Radians to Degrees1/1 -> Steering/1
  Radians to Degrees/1 -> Steering/2
  LiDAR Steering/2(LiDAR Steering) -> Manual Switch2/1, Radians to Degrees/1
  Manual Switch2/1 -> Gain4/1
  Manual Switch1/1 -> Gain2/1
  Square/1 -> Sum1/1
  Second-Order Low-Pass Filter/2 -> Square/1, xy_dot/1
  [xy] -> xy signal maker/2(xy), xy/1
  xy signal maker/1(Out1) -> XY Plot/1
  Constant1/1 -> Second-Order Low-Pass Filter/2
  Signed Sqrt/1 -> speed/1
  Sum1/1 -> Signed Sqrt/1
  [xy_cmd] -> xy signal maker/1(In1)
  Constant2/1 -> Second-Order Low-Pass Filter/3
  [xy] -> Second-Order Low-Pass Filter/1, Second-Order Low-Pass Filter/4
  xy signal maker/2(Out2) -> XY Plot/2
  Saturation/1 -> [Steering], Steering Command/1
  Stop Sign/1 -> MATLAB Function2/2(Stop_Sign)
  Constant10/1 -> MATLAB Function2/3(Sign_Time)
  MATLAB Function2/2(Speed_Multiplier) -> Product/2
  Memory6/1 -> MATLAB Function2/6(Previous_Timer)
  Constant7/1 -> MATLAB Function2/4(No_Sign_Time)
  MATLAB Function2/1(Sign_State) -> Memory7/1
  MATLAB Function2/3(Timer) -> Memory6/1
  Memory7/1 -> MATLAB Function2/1(Previous_State)
  Constant9/1 -> MATLAB Function2/5(Step_size)
  Desired Speed/1 -> Adaptive Cruise Control/2(Desired Speed)
  Gain4/1 -> Sum3/2
  Sum4/1 -> Saturation/1
  Gain2/1 -> Sum3/1
  Constant5/1 -> Second-Order Low-Pass Filter1/3
  Second-Order Low-Pass Filter1/2 -> Gain5/1
  Sum3/1 -> Second-Order Low-Pass Filter1/1, Second-Order Low-Pass Filter1/4, Sum4/1
  Gain5/1 -> Sum4/2
  Constant6/1 -> Second-Order Low-Pass Filter1/2
  [mod_heading] -> Memory1/1
  Path Commander/1(xy_cmd) -> LiDAR Steering/1(xy_command), [xy_cmd]
  Selector/1 -> [xy]
  Position/1 -> Selector/1, Selector1/1
  Selector1/1 -> [mod_heading]
  [xy] -> Path Commander/2(xy)
  Switch/1 -> Path Commander/1(path)
  Path Commander/2(Path_Options) -> Path_Options/1
  Bias1/1 -> Path Commander/3(look_ahead_d)
  Gain1/1 -> Bias1/1
  Speed/1 -> Gain1/1
  Distance to closest car ahead/1 -> Adaptive Cruise Control/1(obstacleDistance (m))
  Clock/1 -> Switch/2
  Path/1 -> Switch/1
  Constant8/1 -> Switch/3
  Subtract/1 -> Traffic Zone 2/3(Traffic Light)
  Traffic Light 1/1 -> Traffic Zone 1/3(Traffic Light), Subtract/2

== system QCar2_Virtual_Car2/Subsystem ==
  Add : Sum
  Data Type Conversion : DataTypeConversion  SaturateOnIntegerOverflow=off  RndMeth=Floor
  Demux : Demux  Outputs=2
  Display : Display
  Display1 : Display
  Gain : Gain
  Gain1 : Gain  Gain=-1
  Host Initialize : quarc_library/Devices/Peripherals/Host/Host Initialize  object_name=Host-1  uri_source=Specify via dialog (do not evaluate)  uri=tcpip://localhost:18002  send_buffer_size=1000  receive_buffer_size=1000  thread_priority=0  run_client=on  use_window=off  window_position=[]  sample_time=qc_get_step_size  active=on
      settings: AttributesFormatString="\"tcpip://localhost:18002\""  SourceProductName=QUARC Targets
  Host Keyboard : quarc_library/Devices/Peripherals/Host/Host Keyboard  object_name=Host-1  virtual_key="[38  40]"  sample_time=qc_get_step_size  enabled=on  debug_mode=off
      settings: SourceProductName=QUARC Targets
  Scope : Scope
  Speed Addition : Outport
  wires:
  Host Keyboard/2 -> Data Type Conversion/1
  Data Type Conversion/1 -> Demux/1, Display/1
  Demux/1 -> Gain/1
  Demux/2 -> Gain1/1
  Gain/1 -> Add/1
  Gain1/1 -> Add/2
  Add/1 -> Speed Addition/1, Scope/1
  Host Keyboard/1 -> Display1/1

== system QCar2_Virtual_Car2/Timing ==
  Computation Time : quarc_library/Sources/Time/Computation Time  sample_time=cameraStepSize  use_model=on  use_cpu_time=off
  Computation Time1 : quarc_library/Sources/Time/Computation Time  sample_time=qc_get_step_size  use_model=on  use_cpu_time=off
  Sample Time : quarc_library/Sources/Time/Sample Time  Priority=-99  sample_time=cameraStepSize
  Sample Time1 : quarc_library/Sources/Time/Sample Time  Priority=-99  sample_time=qc_get_step_size
  Sample_time base : Scope  NumInputPorts=2
  Sample_time camera : Scope  NumInputPorts=2
  wires:
  Computation Time/1 -> Sample_time camera/2
  Sample Time/1 -> Sample_time camera/1
  Sample Time1/1 -> Sample_time base/1
  Computation Time1/1 -> Sample_time base/2
